simulink model "mechanicalSystmes"  (R2021a)
settings: Solver=VariableStepAuto  StartTime=0.0  StopTime=10  FixedStep=0.001  RelTol=1e-3
model workspace (MAT data in the model file):
  b = Simulink.Parameter
  b.Value = 1
  b.DataType = 'int8'
  b.Dimensions = [1 1]
  k = Simulink.Parameter
  k.Value = 4
  k.DataType = 'int8'
  k.Dimensions = [1 1]
  m = Simulink.Parameter
  m.Value = 1
  m.DataType = 'int8'
  m.Dimensions = [1 1]
libraries: slctrlblks x1
settings Model: Creator=User  LastModifiedBy=User
settings OptimizationCC: DefaultParameterBehavior=Inlined  EnhancedBackFolding=on  PassReuseOutputArgsAs=Individual arguments  ZeroExternalMemoryAtStartup=off  ZeroInternalMemoryAtStartup=off  OptimizeBlockOrder=speed  DifferentSizesBufferReuse=on  OptimizationCustomize=off  EfficientTunableParamExpr=on
settings DebuggingCC: ParameterTunabilityLossMsg=error
settings SFSimCC: MATLABDynamicMemAlloc=off
settings RTWCC: SystemTargetFile=ert.tlc  TemplateMakefile=ert_default_tmf
settings CodeAppCC: ForceParamTrailComments=on  IgnoreCustomStorageClasses=off  OperatorAnnotations=on  SimulinkDataObjDesc=on  SFDataObjDesc=on  InsertBlockDesc=on
settings ERTTargetCC: TargetLangStandard=C99 (ISO)  GenerateSampleERTMain=on  InlinedParameterPlacement=NonHierarchical  ERTCustomFileTemplate=example_file_process.tlc
settings ConfigComp: CovEnable=on  CovScope=ReferencedModels  CovIncludeTopModel=off  CovMetricSettings=dcmwe  CovModelRefEnable=filtered

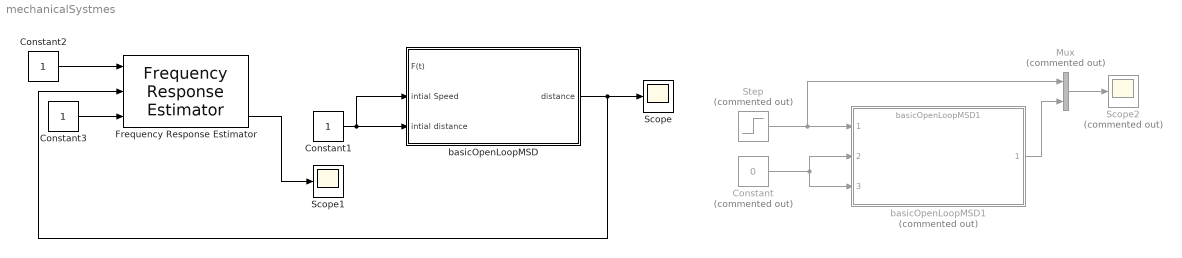
== system mechanicalSystmes ==
  Constant : Constant  Commented=on  Value=0
  Constant1 : Constant
  Constant2 : Constant
  Constant3 : Constant
  Frequency Response Estimator : slctrlblks/Frequency Response Estimator  DiscreteTs=0.1  OutputMode=control action + perturbation  BlockDataType=double  SineSource=Block parameters  Frequencies=[0.5 1 2]  FreqUnits=rad/s  Amplitudes=1  NumOfFreq=3  ExperimentMode=Sinestream  NumOfSetPeriod=2  NumOfEstPeriod=4  NumOfSlowestPeriod=3  EstimationMode=Online  UseBodePlot=off  BaselinePlant=[]  PlotRefreshFactor=100  BodePlotChoice=VariantNull  ExperimentChoice=VariantSS  OutputChoice=VariantCandD
      settings: SourceProductBaseCode=SD
  Mux : Mux  Commented=on  Inputs=2
  Scope : Scope
  Scope1 : Scope
  Scope2 : Scope  Commented=on
  Step : Step  Commented=on  SampleTime=0
  basicOpenLoopMSD : Subsystem  TreatAsAtomicUnit=on
  basicOpenLoopMSD1 : ModelReference  Commented=on  ModelNameDialog=basicOpenLoopMSD1  SimulationMode=Normal  ModelReferenceVersion=1.7
  wires:
  Constant1/1 -> basicOpenLoopMSD/2(intial Speed), basicOpenLoopMSD/3(intial distance)
  basicOpenLoopMSD/1(distance) -> Frequency Response Estimator/2, Scope/1
  Constant2/1 -> Frequency Response Estimator/1
  Frequency Response Estimator/3 -> Scope1/1
  Constant3/1 -> Frequency Response Estimator/3
  Mux/1 -> Scope2/1
  basicOpenLoopMSD1/1 -> Mux/2
  Step/1 -> Mux/1, basicOpenLoopMSD1/1
  Constant/1 -> basicOpenLoopMSD1/3, basicOpenLoopMSD1/2

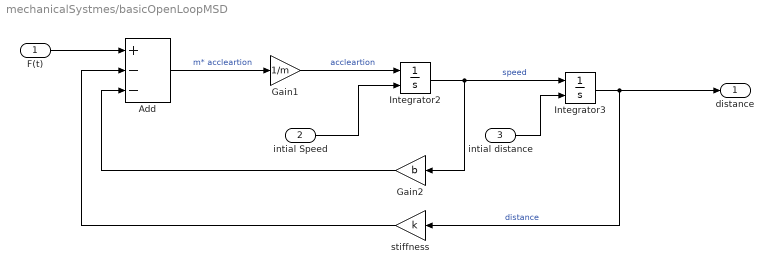
== system mechanicalSystmes/basicOpenLoopMSD ==
  F(t) : Inport
  intial Speed : Inport  Port=2
  intial distance : Inport  Port=3
  Add : Sum  Inputs=+--
  Gain1 : Gain  Gain=1/m
  Gain2 : Gain  Gain=b
  Integrator2 : Integrator  InitialConditionSource=external
  Integrator3 : Integrator  InitialConditionSource=external
  stiffness : Gain  Gain=k
  distance : Outport
  wires:
  intial Speed/1 -> Integrator2/2
  Integrator2/1 -> Integrator3/1, Gain2/1  "speed"
  Gain1/1 -> Integrator2/1  "accleartion"
  intial distance/1 -> Integrator3/2
  Add/1 -> Gain1/1  "m* accleartion"
  Gain2/1 -> Add/3
  stiffness/1 -> Add/2
  Integrator3/1 -> distance/1, stiffness/1  "distance"
  F(t)/1 -> Add/1
